simulink model "robot_etu"  (R2019a)
settings: Solver=VariableStepAuto  StartTime=0.0  StopTime=10.0  RelTol=1e-3
values from neighbouring files (symbols this model uses):
  K = -place(A,B,poles)    [matrices.m]    (also in simu_robot_etu.m = [0.6700,19.9055,1.0747,1.9614])
  ue = 0    [simu_robot_etu.m]
  x0 = [0 pi/10 0 0]'    [simu_robot_etu.m]
  xe = [0 0 0 0]'    [simu_robot_etu.m]
settings Model: Creator=nravalos  LastModifiedBy=nravalos

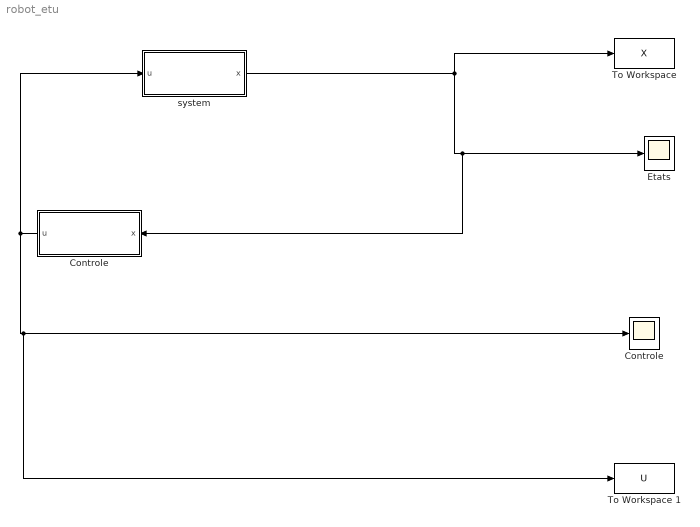
== system robot_etu ==
  Controle : Subsystem
  "Controle " : Scope
  Etats : Scope
  "To Workspace " : ToWorkspace  VariableName=X  SaveFormat=Timeseries  SampleTime=-1
  "To Workspace 1 " : ToWorkspace  VariableName=U  SaveFormat=Timeseries  SampleTime=-1
  system : Subsystem
  wires:
  system/1(x) -> Controle/1(x), Etats/1, "To Workspace "/1
  Controle/1(u) -> system/1("u "), "To Workspace 1 "/1, "Controle "/1

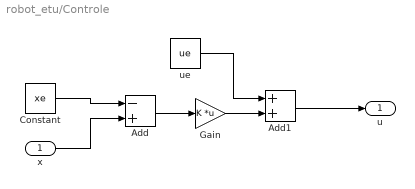
== system robot_etu/Controle ==
  x : Inport
  Add : Sum  Inputs=-+
  Add1 : Sum
  Constant : Constant  Value=xe
  Gain : Gain  Gain=K  Multiplication=Matrix(K*u)
  ue : Constant  Value=ue
  u : Outport
  wires:
  x/1 -> Add/2
  Add1/1 -> u/1
  ue/1 -> Add1/1
  Gain/1 -> Add1/2
  Constant/1 -> Add/1
  Add/1 -> Gain/1

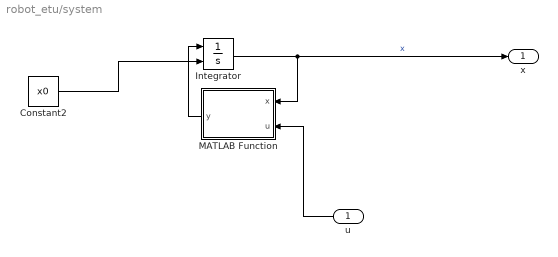
== system robot_etu/system ==
  "u " : Inport
  Constant2 : Constant  Value=x0
  Integrator : Integrator  InitialConditionSource=external
  MATLAB Function : MATLAB Function  TreatAsAtomicUnit=on
  x : Outport
  wires:
  "u "/1 -> MATLAB Function/2(u)
  Integrator/1 -> x/1, MATLAB Function/1(x)  "x"
  MATLAB Function/1(y) -> Integrator/1
  Constant2/1 -> Integrator/2

== matlab function robot_etu/system/MATLAB Function ==
  data: x input; u input; y output
function y = fcn(x, u)

y = fonction(x,u);
